simulink model "clk"  (R2017a)
settings: Solver=VariableStepAuto  StartTime=0.0  StopTime=10.0  RelTol=1e-3
values from neighbouring files (symbols this model uses):
  dtheta1_throw_traj = linspace(0, 1, 10)    [ballToss.m]
  dtheta2_throw_traj = linspace(0, 1, 10)    [ballToss.m]
  theta1_init_traj = linspace(0, 1, 10)    [ballToss.m]
  theta1_throw_traj = linspace(0, 1, 10)    [ballToss.m]
  theta2_init_traj = linspace(0, 1, 10)    [ballToss.m]
  theta2_throw_traj = linspace(0, 1, 10)    [ballToss.m]
undefined symbols (not defined in the file or in its folder): Ts_traj, Ts_traj_throw
settings Model: Creator=sondrebk  LastModifiedBy=sondrebk

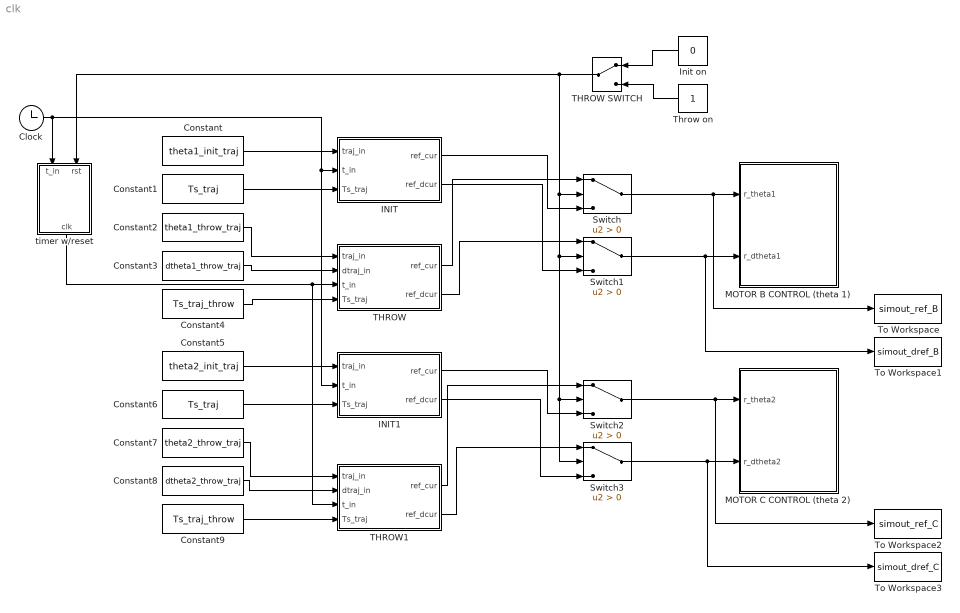
== system clk ==
  Clock : Clock
  Constant : Constant  Value=theta1_init_traj
  Constant1 : Constant  Value=Ts_traj
  Constant2 : Constant  Value=theta1_throw_traj
  Constant3 : Constant  Value=dtheta1_throw_traj
  Constant4 : Constant  Value=Ts_traj_throw
  Constant5 : Constant  Value=theta2_init_traj
  Constant6 : Constant  Value=Ts_traj
  Constant7 : Constant  Value=theta2_throw_traj
  Constant8 : Constant  Value=dtheta2_throw_traj
  Constant9 : Constant  Value=Ts_traj_throw
  INIT : MATLAB Function  TreatAsAtomicUnit=on
  INIT1 : MATLAB Function  TreatAsAtomicUnit=on
  Init on : Constant  Value=0
  MOTOR B CONTROL (theta 1) : Subsystem
  MOTOR C CONTROL (theta 2) : Subsystem
  Switch{,1..3} (4 alike) : Switch  Criteria=u2 > Threshold
  THROW : MATLAB Function  TreatAsAtomicUnit=on
  THROW SWITCH : ManualSwitch
  THROW1 : MATLAB Function  TreatAsAtomicUnit=on
  Throw on : Constant
  To Workspace : ToWorkspace  VariableName=simout_ref_B  SaveFormat=Timeseries  SampleTime=-1
  To Workspace1 : ToWorkspace  VariableName=simout_dref_B  SaveFormat=Timeseries  SampleTime=-1
  To Workspace2 : ToWorkspace  VariableName=simout_ref_C  SaveFormat=Timeseries  SampleTime=-1
  To Workspace3 : ToWorkspace  VariableName=simout_dref_C  SaveFormat=Timeseries  SampleTime=-1
  timer w/reset : MATLAB Function  TreatAsAtomicUnit=on
  wires:
  Throw on/1 -> THROW SWITCH/2
  Init on/1 -> THROW SWITCH/1
  THROW SWITCH/1 -> timer w/reset/2(rst), Switch3/2, Switch2/2, Switch1/2, Switch/2
  Switch1/1 -> To Workspace1/1, MOTOR B CONTROL (theta 1)/2(r_dtheta1)
  Switch/1 -> To Workspace/1, MOTOR B CONTROL (theta 1)/1(r_theta1)
  Switch2/1 -> To Workspace2/1, MOTOR C CONTROL (theta 2)/1(r_theta2)
  Switch3/1 -> To Workspace3/1, MOTOR C CONTROL (theta 2)/2(r_dtheta2)
  INIT/1(ref_cur) -> Switch/3
  THROW/1(ref_cur) -> Switch/1
  INIT/2(ref_dcur) -> Switch1/3
  THROW/2(ref_dcur) -> Switch1/1
  Constant/1 -> INIT/1(traj_in)
  Clock/1 -> timer w/reset/1(t_in), INIT1/2(t_in), INIT/2(t_in)
  timer w/reset/1(clk) -> THROW/3(t_in), THROW1/3(t_in)
  Constant1/1 -> INIT/3(Ts_traj)
  Constant2/1 -> THROW/1(traj_in)
  Constant3/1 -> THROW/2(dtraj_in)
  Constant4/1 -> THROW/4(Ts_traj)
  Constant7/1 -> THROW1/1(traj_in)
  Constant8/1 -> THROW1/2(dtraj_in)
  Constant9/1 -> THROW1/4(Ts_traj)
  Constant5/1 -> INIT1/1(traj_in)
  Constant6/1 -> INIT1/3(Ts_traj)
  THROW1/2(ref_dcur) -> Switch3/1
  INIT1/2(ref_dcur) -> Switch3/3
  THROW1/1(ref_cur) -> Switch2/1
  INIT1/1(ref_cur) -> Switch2/3

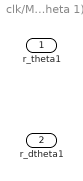
== system clk/MOTOR B CONTROL (theta 1) ==
  r_theta1 : Inport
  r_dtheta1 : Inport  Port=2

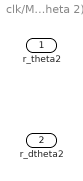
== system clk/MOTOR C CONTROL (theta 2) ==
  r_theta2 : Inport
  r_dtheta2 : Inport  Port=2

== matlab function clk/INIT ==
  data: traj_in input; ref_cur output; t_in input; Ts_traj input; ref_dcur output
function [ref_cur, ref_dcur] = fcn(traj_in, t_in, Ts_traj)

ref_cur = 1;
ref_dcur = 1;

== matlab function clk/timer w//reset ==
  data: t_in input; clk output; rst input
function clk = fcn(t_in, rst)
persistent t_off last_rst
if isempty(t_off)
    t_off = 0;
end
if isempty(last_rst)
    last_rst = 0;
end

% if rest switch was pressed, use current time as t_offset
if abs(rst - last_rst) ~= 0
    t_off = t_in;
end

clk = t_in - t_off; % output clock
last_rst = rst;     % update reset var

== matlab function clk/THROW ==
  data: traj_in input; dtraj_in input; ref_cur output; t_in input; Ts_traj input; ref_dcur output
function [ref_cur, ref_dcur] = fcn(traj_in, dtraj_in, t_in, Ts_traj)

ref_cur = 1;
ref_dcur = 1;

== matlab function clk/INIT1 ==
  data: traj_in input; ref_cur output; t_in input; Ts_traj input; ref_dcur output
function [ref_cur, ref_dcur] = fcn(traj_in, t_in, Ts_traj)

ref_cur = 1;
ref_dcur = 1;

== matlab function clk/THROW1 ==
  data: traj_in input; dtraj_in input; ref_cur output; t_in input; Ts_traj input; ref_dcur output
function [ref_cur, ref_dcur] = fcn(traj_in, dtraj_in, t_in, Ts_traj)

ref_cur = 1;
ref_dcur = 1;
